simulink model "test_v2"  (R2019b)
settings: Solver=ode4  StartTime=0.0  StopTime=300  FixedStep=0.0005
libraries: simulink x3, dspsrcs4 x1
settings Model: Creator=bitgar  LastModifiedBy=bitgar

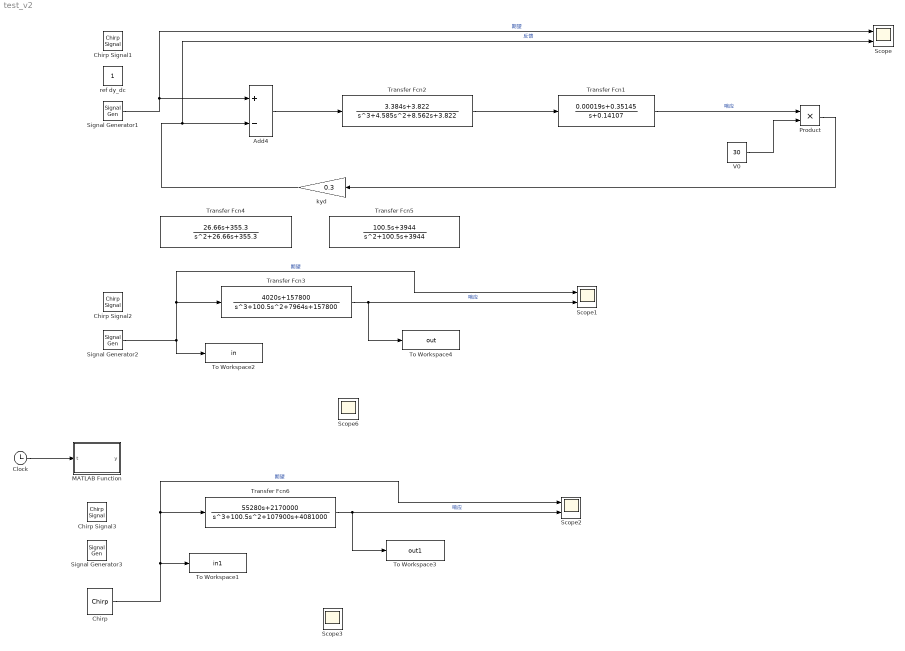
== system test_v2 ==
  Add4 : Sum  Inputs=+-
  Chirp : dspsrcs4/Chirp  sweep=Logarithmic  mode=Unidirectional  f0=0.1  f1=150  t1=300  Tsweep=300  phase=1.5*pi  Ts=0.0005  spf=1  datatype=Double  OutputFrames=off
      settings: SourceProductName=DSP System Toolbox
  Chirp Signal1 : simulink/Sources/Chirp Signal  f1=0.001  T=100  f2=2.5
  Chirp Signal2 : simulink/Sources/Chirp Signal  f1=0.001  T=100  f2=2.5
  Chirp Signal3 : simulink/Sources/Chirp Signal  f1=0.001  T=500  f2=300
  Clock : Clock
  MATLAB Function : MATLAB Function  TreatAsAtomicUnit=on
  Product : Product
  Scope{,1..3,6} (5 alike) : Scope  NumInputPorts=2
  Signal Generator1 : SignalGenerator  Frequency=0.0334
  Signal Generator2 : SignalGenerator  Frequency=3
  Signal Generator3 : SignalGenerator  Frequency=3
  To Workspace1 : ToWorkspace  VariableName=in1  SampleTime=-1
      settings: Save2DSignal=2-D array (concatenate along first dimension)
  To Workspace2 : ToWorkspace  VariableName=in  SampleTime=-1
  To Workspace3 : ToWorkspace  VariableName=out1  SampleTime=-1
      settings: Save2DSignal=2-D array (concatenate along first dimension)
  To Workspace4 : ToWorkspace  VariableName=out  SampleTime=-1
  Transfer Fcn1 : TransferFcn  Numerator=[0.00019 0.35145]  Denominator=[1 0.14107]
  Transfer Fcn2 : TransferFcn  Numerator=[3.384 3.822]  Denominator=[1 4.585 8.562 3.822]
  Transfer Fcn3 : TransferFcn  Numerator=[4020 157800]  Denominator=[1 100.5 7964 157800]
  Transfer Fcn4 : TransferFcn  Numerator=[26.66 355.3]  Denominator=[1 26.66 355.3]
  Transfer Fcn5 : TransferFcn  Numerator=[100.5 3944]  Denominator=[1 100.5 3944]
  Transfer Fcn6 : TransferFcn  Numerator=[55280 2170000]  Denominator=[1 100.5 107900 4081000]
  V0 : Constant  Value=30
  kyd : Gain  Gain=0.3
  ref dy_dc : Constant
  wires:
  ? -> ?
  Transfer Fcn1/1 -> Product/1  "响应"
  Signal Generator1/1 -> Scope/1, Add4/1  "期望"
  kyd/1 -> Add4/2, Scope/2  "反馈"
  V0/1 -> Product/2
  Product/1 -> kyd/1
  Add4/1 -> Transfer Fcn2/1
  Transfer Fcn2/1 -> Transfer Fcn1/1
  Signal Generator2/1 -> Scope1/1, Transfer Fcn3/1, To Workspace2/1  "期望"
  Transfer Fcn3/1 -> To Workspace4/1, Scope1/2  "响应"
  Transfer Fcn6/1 -> To Workspace3/1, Scope2/2  "响应"
  Chirp/1 -> Scope2/1, Transfer Fcn6/1, To Workspace1/1  "期望"
  Clock/1 -> MATLAB Function/1(t)

== matlab function test_v2/MATLAB Function ==
  data: t input; y output
function y = fcn(t)
    % --- 参数设置 ---
    f0 = 0.1;   % 起始频率 (Hz) -> 覆盖低频零点 (6Hz)
    f1 = 150;   % 终止频率 (Hz) -> 覆盖共振峰 (52Hz) 并留出衰减余量
    T  = 300;   % 扫频时间 (s)  -> 300秒足够慢，能保证能量充足
    % ----------------
    
    % 对数扫频公式 (Logarithmic Chirp Instantaneous Phase)
    % 这里的公式对应的是频率随时间指数增长
    
    if t <= T
        % β = T / ln(f1/f0)
        beta = T / log(f1/f0);
        
        % 相位积分 Result: 2*pi * f0 * beta * ((f1/f0)^(t/T) - 1)
        phase = 2 * pi * f0 * beta * ( (f1/f0)^(t/T) - 1 );
        
        y = sin(phase);
    else
        % 扫频结束后归零，或者保持最后频率 sin(phase_end + ...)
        y = 0; 
    end
end
